simulink model "Multi_agent_system"  (R2016b)
settings: Solver=VariableStepAuto  StartTime=0.0  StopTime=100  RelTol=1e-3
undefined symbols (not defined in the file or in its folder): F, L, n, P, v_initial, x_hat_initial, x_initial
settings Model: Creator=kvlton  LastModifiedBy=kvlton

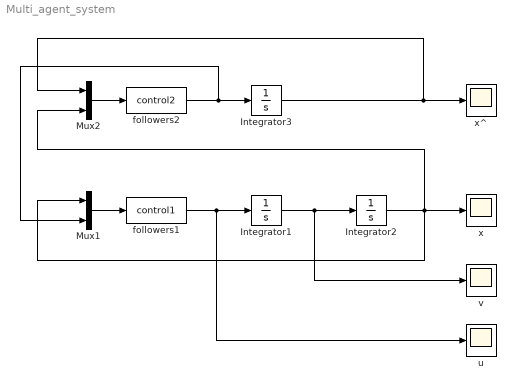
== system Multi_agent_system ==
  Integrator1 : Integrator  InitialCondition=v_initial
  Integrator2 : Integrator  InitialCondition=x_initial
  Integrator3 : Integrator  InitialCondition=x_hat_initial
  Mux1 : Mux  Inputs=2
  Mux2 : Mux  Inputs=2
  followers1 : S-Function  FunctionName=control1  Parameters=L,P,n  SFunctionDeploymentMode=off  EnableBusSupport=off
  followers2 : S-Function  FunctionName=control2  Parameters=F,L,n  SFunctionDeploymentMode=off  EnableBusSupport=off
  u : Scope
  v : Scope
  x : Scope
  x^ : Scope
  wires:
  Mux1/1 -> followers1/1
  followers1/1 -> u/1, Integrator1/1
  Integrator1/1 -> v/1, Integrator2/1
  Integrator2/1 -> Mux1/1, Mux2/2, x/1
  Integrator3/1 -> Mux2/1, x^/1
  followers2/1 -> Mux1/2, Integrator3/1
  Mux2/1 -> followers2/1
